simulink model "Exercicio_1_sim"  (R2016a)
settings: Solver=VariableStepAuto  StartTime=0.0  StopTime=t_sim  RelTol=1e-3
values from neighbouring files (symbols this model uses):
  A = [[0,1,0];[0,0,1];[-0.005,-0.11,-0.7]]    [Exercicio_1.m]    (also in matlab.mat = [0  1  0; 0  0  1; -0.005  -0.11  -0.7])
  A2 = [[-0.2,-0.2,0.4];[0.5,0,1];[0,-0.4,-0.4]]    [Exercicio_1.m]    (also in matlab.mat = [-0.2  -0.2  0.4; 0.5  0  1; 0  -0.4  -0.4])
  Aobs_A1 = A    [Exercicio_1.m]    (also in matlab.mat = [0  1  0; 0  0  1; -0.005  -0.11  -0.7])
  Aobs_B1 = A2    [Exercicio_1.m]    (also in matlab.mat = [-0.2  -0.2  0.4; 0.5  0  1; 0  -0.4  -0.4])
  B = [[0.1];[-0.2];[-0.1]]    [Exercicio_1.m]    (also in matlab.mat = [0.1 -0.2 -0.1])
  B2 = [[0.01];[0];[0.05]]    [Exercicio_1.m]    (also in matlab.mat = [0.01 0 0.05])
  Bobs_A1 = B    [Exercicio_1.m]    (also in matlab.mat = [0.1 -0.2 -0.1])
  Bobs_B1 = B2    [Exercicio_1.m]    (also in matlab.mat = [0.01 0 0.05])
  C = [0,0,1]    [Exercicio_1.m]    (also in matlab.mat = [0 0 1])
  C2 = [1,0,0]    [Exercicio_1.m]    (also in matlab.mat = [1 0 0])
  Cobs_A1 = C    [Exercicio_1.m]    (also in matlab.mat = [0 0 1])
  Cobs_B1 = C2    [Exercicio_1.m]    (also in matlab.mat = [1 0 0])
  D = [0]    [Exercicio_1.m]    (also in matlab.mat = 0)
  D2 = [0]    [Exercicio_1.m]    (also in matlab.mat = 0)
  Dobs_A1 = D    [Exercicio_1.m]    (also in matlab.mat = 0)
  Dobs_B1 = D2    [Exercicio_1.m]    (also in matlab.mat = 0)
  Keobs_A1 = [(Ke1_A1);(Ke2_A1);(Ke3_A1)]    [Exercicio_1.m]    (also in matlab.mat = [87026 -4185 9.81])
  Keobs_B1 = [(Ke1_B1);(Ke2_B1);(Ke3_B1)]    [Exercicio_1.m]    (also in matlab.mat = [8.18 -42.462 15.264])
settings Model: Creator=Usuario  LastModifiedBy=Eletrônica Auto Poli

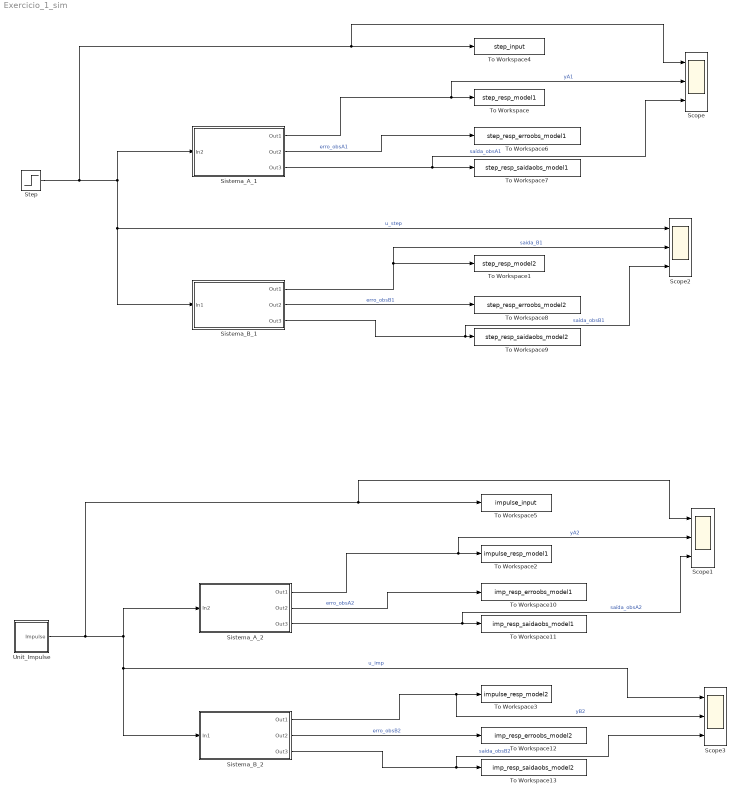
== system Exercicio_1_sim ==
  Scope{,1..3} (4 alike) : Scope  NumInputPorts=3
  Sistema_A_1 : Subsystem
  Sistema_A_2 : Subsystem
  Sistema_B_1 : Subsystem
  Sistema_B_2 : Subsystem
  Step : Step  SampleTime=0.01
  To Workspace : ToWorkspace  VariableName=step_resp_model1  SaveFormat=Timeseries  SampleTime=-1
  To Workspace1 : ToWorkspace  VariableName=step_resp_model2  SaveFormat=Timeseries  SampleTime=-1
  To Workspace10 : ToWorkspace  VariableName=imp_resp_erroobs_model1  SaveFormat=Timeseries  SampleTime=-1
  To Workspace11 : ToWorkspace  VariableName=imp_resp_saidaobs_model1  SaveFormat=Timeseries  SampleTime=-1
  To Workspace12 : ToWorkspace  VariableName=imp_resp_erroobs_model2  SaveFormat=Timeseries  SampleTime=-1
  To Workspace13 : ToWorkspace  VariableName=imp_resp_saidaobs_model2  SaveFormat=Timeseries  SampleTime=-1
  To Workspace2 : ToWorkspace  VariableName=impulse_resp_model1  SaveFormat=Timeseries  SampleTime=-1
  To Workspace3 : ToWorkspace  VariableName=impulse_resp_model2  SaveFormat=Timeseries  SampleTime=-1
  To Workspace4 : ToWorkspace  VariableName=step_input  SaveFormat=Timeseries  SampleTime=-1
  To Workspace5 : ToWorkspace  VariableName=impulse_input  SaveFormat=Timeseries  SampleTime=-1
  To Workspace6 : ToWorkspace  VariableName=step_resp_erroobs_model1  SaveFormat=Timeseries  SampleTime=-1
  To Workspace7 : ToWorkspace  VariableName=step_resp_saidaobs_model1  SaveFormat=Timeseries  SampleTime=-1
  To Workspace8 : ToWorkspace  VariableName=step_resp_erroobs_model2  SaveFormat=Timeseries  SampleTime=-1
  To Workspace9 : ToWorkspace  VariableName=step_resp_saidaobs_model2  SaveFormat=Timeseries  SampleTime=-1
  Unit_Impulse : Subsystem
  wires:
  Step/1 -> Scope/1, To Workspace4/1, Sistema_A_1/1(In2), Scope2/1, Sistema_B_1/1(In1)  "u_step"
  Sistema_A_1/1(Out1) -> Scope/2, To Workspace/1  "yA1"
  Sistema_A_1/2(Out2) -> To Workspace6/1  "erro_obsA1"
  Sistema_A_1/3(Out3) -> Scope/3, To Workspace7/1  "saída_obsA1"
  Sistema_B_1/2(Out2) -> To Workspace8/1  "erro_obsB1"
  Unit_Impulse/1(Impulse) -> Scope1/1, To Workspace5/1, Sistema_A_2/1(In2), Scope3/1, Sistema_B_2/1(In1)  "u_imp"
  Sistema_A_2/1(Out1) -> Scope1/2, To Workspace2/1  "yA2"
  Sistema_B_2/1(Out1) -> Scope3/2, To Workspace3/1  "yB2"
  Sistema_A_2/2(Out2) -> To Workspace10/1  "erro_obsA2"
  Sistema_A_2/3(Out3) -> Scope1/3, To Workspace11/1  "saída_obsA2"
  Sistema_B_2/2(Out2) -> To Workspace12/1  "erro_obsB2"
  Sistema_B_2/3(Out3) -> Scope3/3, To Workspace13/1  "saída_obsB2"
  Sistema_B_1/1(Out1) -> To Workspace1/1, Scope2/2  "saida_B1"
  Sistema_B_1/3(Out3) -> Scope2/3, To Workspace9/1  "saída_obsB1"

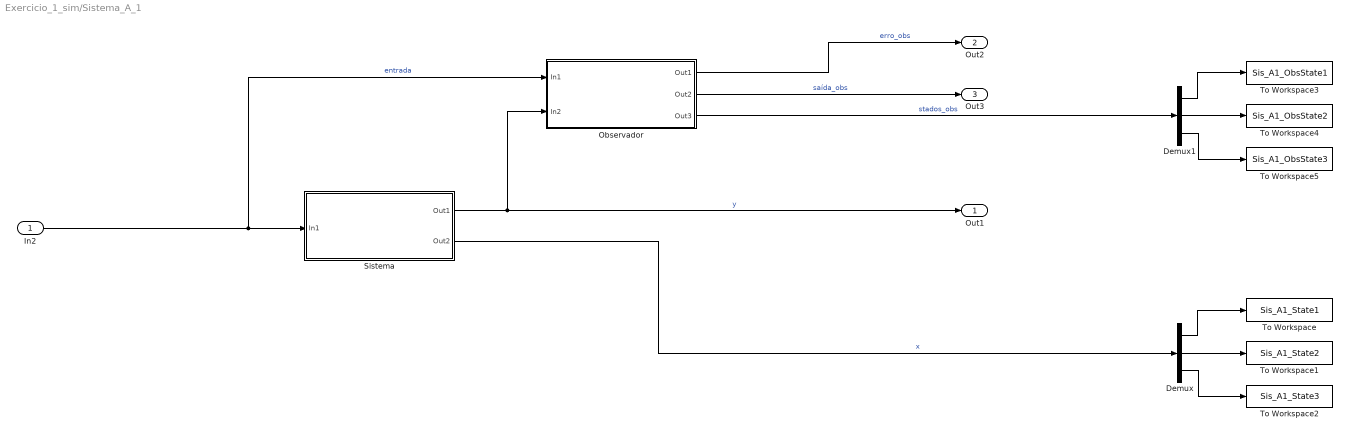
== system Exercicio_1_sim/Sistema_A_1 ==
  In2 : Inport
  Demux : Demux  Outputs=3
  Demux1 : Demux  Outputs=3
  Observador : Subsystem
  Sistema : Subsystem
  To Workspace : ToWorkspace  VariableName=Sis_A1_State1  SaveFormat=Timeseries  SampleTime=-1
  To Workspace1 : ToWorkspace  VariableName=Sis_A1_State2  SaveFormat=Timeseries  SampleTime=-1
  To Workspace2 : ToWorkspace  VariableName=Sis_A1_State3  SaveFormat=Timeseries  SampleTime=-1
  To Workspace3 : ToWorkspace  VariableName=Sis_A1_ObsState1  SaveFormat=Timeseries  SampleTime=-1
  To Workspace4 : ToWorkspace  VariableName=Sis_A1_ObsState2  SaveFormat=Timeseries  SampleTime=-1
  To Workspace5 : ToWorkspace  VariableName=Sis_A1_ObsState3  SaveFormat=Timeseries  SampleTime=-1
  Out1 : Outport
  Out2 : Outport  Port=2
  Out3 : Outport  Port=3
  wires:
  Demux/1 -> To Workspace/1
  Demux/2 -> To Workspace1/1
  Demux/3 -> To Workspace2/1
  In2/1 -> Observador/1(In1), Sistema/1(In1)  "entrada"
  Sistema/1(Out1) -> Out1/1, Observador/2(In2)  "y"
  Sistema/2(Out2) -> Demux/1  "x"
  Demux1/1 -> To Workspace3/1
  Demux1/2 -> To Workspace4/1
  Demux1/3 -> To Workspace5/1
  Observador/1(Out1) -> Out2/1  "erro_obs"
  Observador/2(Out2) -> Out3/1  "saída_obs"
  Observador/3(Out3) -> Demux1/1  "stados_obs"

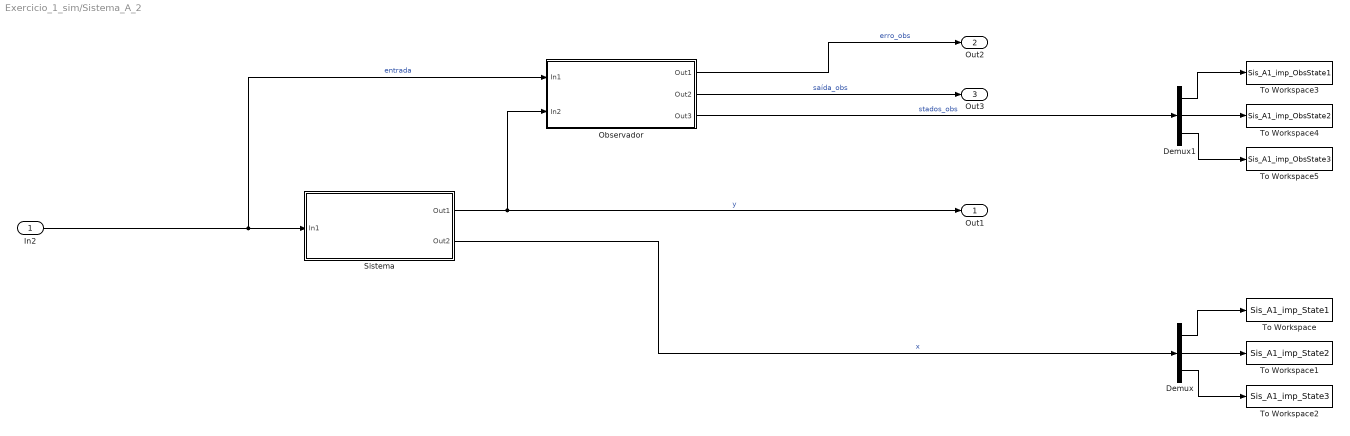
== system Exercicio_1_sim/Sistema_A_2 ==
  In2 : Inport
  Demux : Demux  Outputs=3
  Demux1 : Demux  Outputs=3
  Observador : Subsystem
  Sistema : Subsystem
  To Workspace : ToWorkspace  VariableName=Sis_A1_imp_State1  SaveFormat=Timeseries  SampleTime=-1
  To Workspace1 : ToWorkspace  VariableName=Sis_A1_imp_State2  SaveFormat=Timeseries  SampleTime=-1
  To Workspace2 : ToWorkspace  VariableName=Sis_A1_imp_State3  SaveFormat=Timeseries  SampleTime=-1
  To Workspace3 : ToWorkspace  VariableName=Sis_A1_imp_ObsState1  SaveFormat=Timeseries  SampleTime=-1
  To Workspace4 : ToWorkspace  VariableName=Sis_A1_imp_ObsState2  SaveFormat=Timeseries  SampleTime=-1
  To Workspace5 : ToWorkspace  VariableName=Sis_A1_imp_ObsState3  SaveFormat=Timeseries  SampleTime=-1
  Out1 : Outport
  Out2 : Outport  Port=2
  Out3 : Outport  Port=3
  wires:
  Demux/1 -> To Workspace/1
  Demux/2 -> To Workspace1/1
  Demux/3 -> To Workspace2/1
  In2/1 -> Observador/1(In1), Sistema/1(In1)  "entrada"
  Sistema/1(Out1) -> Out1/1, Observador/2(In2)  "y"
  Sistema/2(Out2) -> Demux/1  "x"
  Demux1/1 -> To Workspace3/1
  Demux1/2 -> To Workspace4/1
  Demux1/3 -> To Workspace5/1
  Observador/1(Out1) -> Out2/1  "erro_obs"
  Observador/2(Out2) -> Out3/1  "saída_obs"
  Observador/3(Out3) -> Demux1/1  "stados_obs"

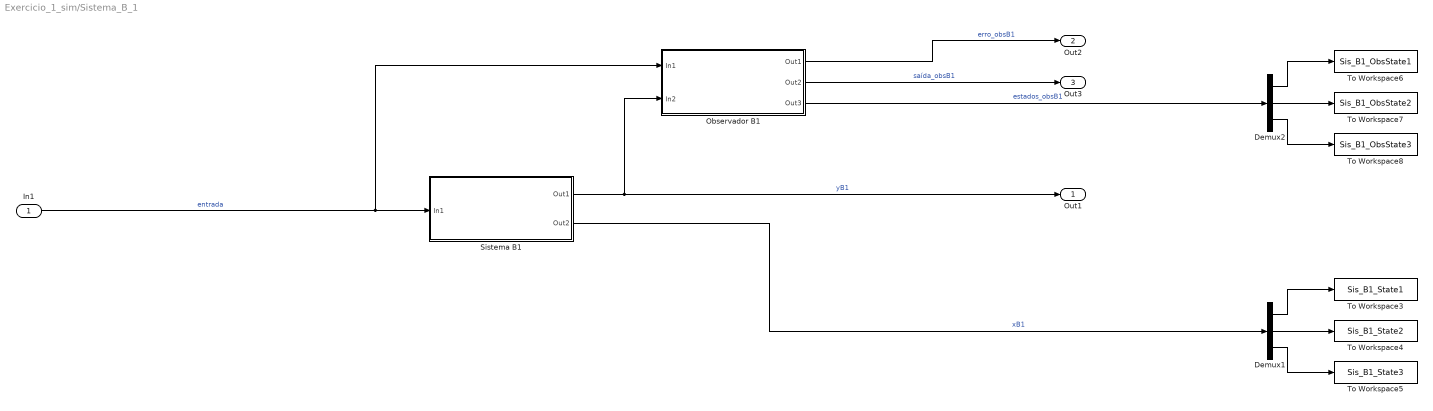
== system Exercicio_1_sim/Sistema_B_1 ==
  In1 : Inport
  Demux1 : Demux  Outputs=3
  Demux2 : Demux  Outputs=3
  Observador B1 : Subsystem
  Sistema B1 : Subsystem
  To Workspace3 : ToWorkspace  VariableName=Sis_B1_State1  SaveFormat=Timeseries  SampleTime=-1
  To Workspace4 : ToWorkspace  VariableName=Sis_B1_State2  SaveFormat=Timeseries  SampleTime=-1
  To Workspace5 : ToWorkspace  VariableName=Sis_B1_State3  SaveFormat=Timeseries  SampleTime=-1
  To Workspace6 : ToWorkspace  VariableName=Sis_B1_ObsState1  SaveFormat=Timeseries  SampleTime=-1
  To Workspace7 : ToWorkspace  VariableName=Sis_B1_ObsState2  SaveFormat=Timeseries  SampleTime=-1
  To Workspace8 : ToWorkspace  VariableName=Sis_B1_ObsState3  SaveFormat=Timeseries  SampleTime=-1
  Out1 : Outport
  Out2 : Outport  Port=2
  Out3 : Outport  Port=3
  wires:
  Demux1/1 -> To Workspace3/1
  Demux1/2 -> To Workspace4/1
  Demux1/3 -> To Workspace5/1
  In1/1 -> Observador B1/1(In1), Sistema B1/1(In1)  "entrada"
  Sistema B1/1(Out1) -> Out1/1, Observador B1/2(In2)  "yB1"
  Sistema B1/2(Out2) -> Demux1/1  "xB1"
  Demux2/1 -> To Workspace6/1
  Demux2/2 -> To Workspace7/1
  Demux2/3 -> To Workspace8/1
  Observador B1/1(Out1) -> Out2/1  "erro_obsB1"
  Observador B1/2(Out2) -> Out3/1  "saída_obsB1"
  Observador B1/3(Out3) -> Demux2/1  "estados_obsB1"

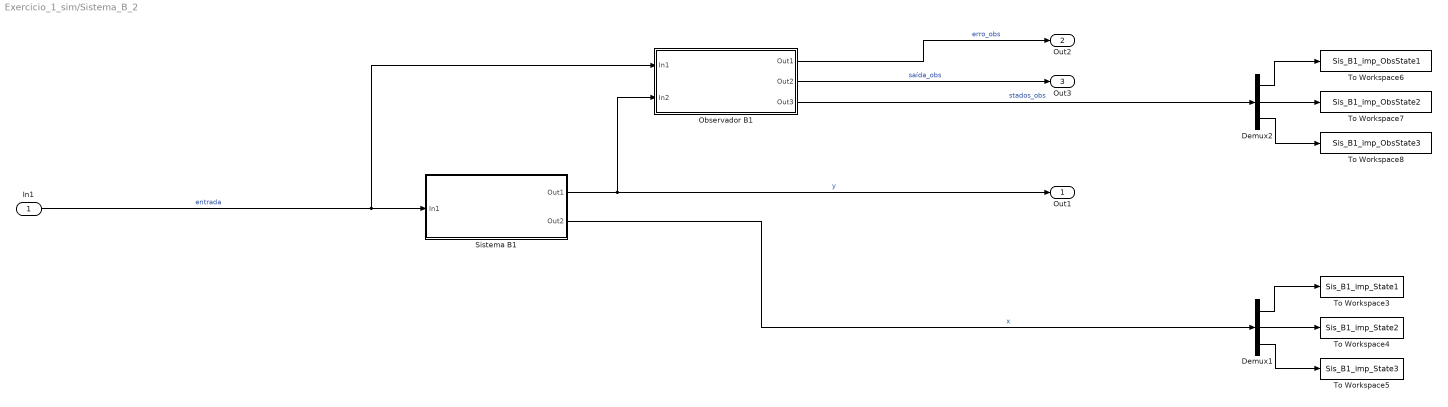
== system Exercicio_1_sim/Sistema_B_2 ==
  In1 : Inport
  Demux1 : Demux  Outputs=3
  Demux2 : Demux  Outputs=3
  Observador B1 : Subsystem
  Sistema B1 : Subsystem
  To Workspace3 : ToWorkspace  VariableName=Sis_B1_imp_State1  SaveFormat=Timeseries  SampleTime=-1
  To Workspace4 : ToWorkspace  VariableName=Sis_B1_imp_State2  SaveFormat=Timeseries  SampleTime=-1
  To Workspace5 : ToWorkspace  VariableName=Sis_B1_imp_State3  SaveFormat=Timeseries  SampleTime=-1
  To Workspace6 : ToWorkspace  VariableName=Sis_B1_imp_ObsState1  SaveFormat=Timeseries  SampleTime=-1
  To Workspace7 : ToWorkspace  VariableName=Sis_B1_imp_ObsState2  SaveFormat=Timeseries  SampleTime=-1
  To Workspace8 : ToWorkspace  VariableName=Sis_B1_imp_ObsState3  SaveFormat=Timeseries  SampleTime=-1
  Out1 : Outport
  Out2 : Outport  Port=2
  Out3 : Outport  Port=3
  wires:
  Demux1/1 -> To Workspace3/1
  Demux1/2 -> To Workspace4/1
  Demux1/3 -> To Workspace5/1
  In1/1 -> Observador B1/1(In1), Sistema B1/1(In1)  "entrada"
  Sistema B1/1(Out1) -> Out1/1, Observador B1/2(In2)  "y"
  Sistema B1/2(Out2) -> Demux1/1  "x"
  Demux2/1 -> To Workspace6/1
  Demux2/2 -> To Workspace7/1
  Demux2/3 -> To Workspace8/1
  Observador B1/1(Out1) -> Out2/1  "erro_obs"
  Observador B1/2(Out2) -> Out3/1  "saída_obs"
  Observador B1/3(Out3) -> Demux2/1  "stados_obs"

== system Exercicio_1_sim/Unit_Impulse ==
  Step1 : Step  Time=0.5  After=100  SampleTime=0.01
  Step2 : Step  Time=0.51  After=100  SampleTime=0.01
  Sum : Sum  Inputs=|+-
  Impulse : Outport
  wires:
  Step2/1 -> Sum/2
  Step1/1 -> Sum/1
  Sum/1 -> Impulse/1

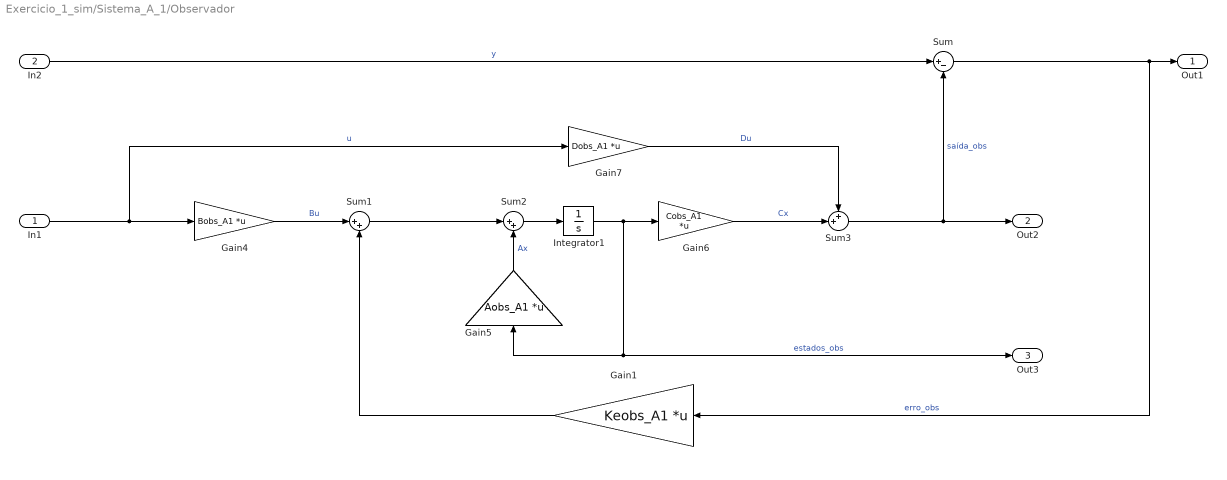
== system Exercicio_1_sim/Sistema_A_1/Observador ==
  In1 : Inport
  In2 : Inport  Port=2
  Gain1 : Gain  Gain=Keobs_A1  Multiplication=Matrix(K*u)
  Gain4 : Gain  Gain=Bobs_A1  Multiplication=Matrix(K*u)
  Gain5 : Gain  Gain=Aobs_A1  Multiplication=Matrix(K*u)
  Gain6 : Gain  Gain=Cobs_A1  Multiplication=Matrix(K*u)
  Gain7 : Gain  Gain=Dobs_A1  Multiplication=Matrix(K*u)
  Integrator1 : Integrator  InitialCondition=[3,7,5]
  Sum : Sum  Inputs=|+-
  Sum1 : Sum  Inputs=|++
  Sum2 : Sum  Inputs=|++
  Sum3 : Sum  Inputs=++|
  Out1 : Outport
  Out2 : Outport  Port=2
  Out3 : Outport  Port=3
  wires:
  Sum3/1 -> Out2/1, Sum/2  "saída_obs"
  Integrator1/1 -> Out3/1, Gain5/1, Gain6/1  "estados_obs"
  Gain6/1 -> Sum3/2  "Cx"
  Gain7/1 -> Sum3/1  "Du"
  Gain4/1 -> Sum1/1  "Bu"
  Gain5/1 -> Sum2/2  "Ax"
  Sum2/1 -> Integrator1/1
  In2/1 -> Sum/1  "y"
  In1/1 -> Gain4/1, Gain7/1  "u"
  Sum/1 -> Out1/1, Gain1/1  "erro_obs"
  Sum1/1 -> Sum2/1
  Gain1/1 -> Sum1/2

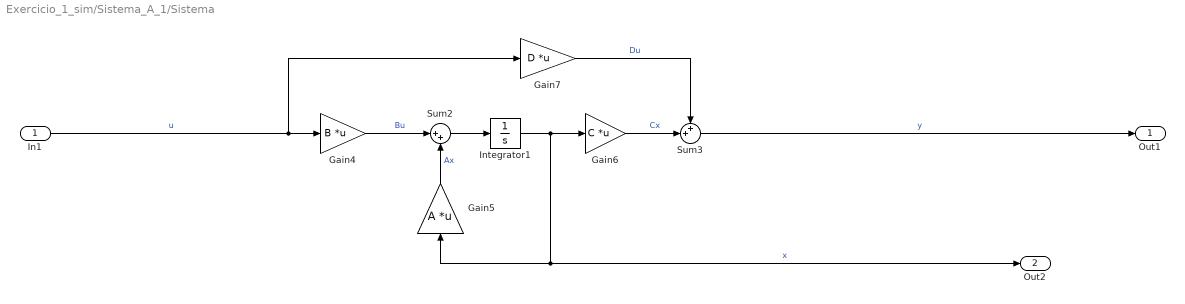
== system Exercicio_1_sim/Sistema_A_1/Sistema ==
  In1 : Inport
  Gain4 : Gain  Gain=B  Multiplication=Matrix(K*u)
  Gain5 : Gain  Gain=A  Multiplication=Matrix(K*u)
  Gain6 : Gain  Gain=C  Multiplication=Matrix(K*u)
  Gain7 : Gain  Gain=D  Multiplication=Matrix(K*u)
  Integrator1 : Integrator
  Sum2 : Sum  Inputs=|++
  Sum3 : Sum  Inputs=++|
  Out1 : Outport
  Out2 : Outport  Port=2
  wires:
  In1/1 -> Gain7/1, Gain4/1  "u"
  Sum3/1 -> Out1/1  "y"
  Integrator1/1 -> Out2/1, Gain5/1, Gain6/1  "x"
  Gain6/1 -> Sum3/2  "Cx"
  Gain7/1 -> Sum3/1  "Du"
  Gain4/1 -> Sum2/1  "Bu"
  Gain5/1 -> Sum2/2  "Ax"
  Sum2/1 -> Integrator1/1

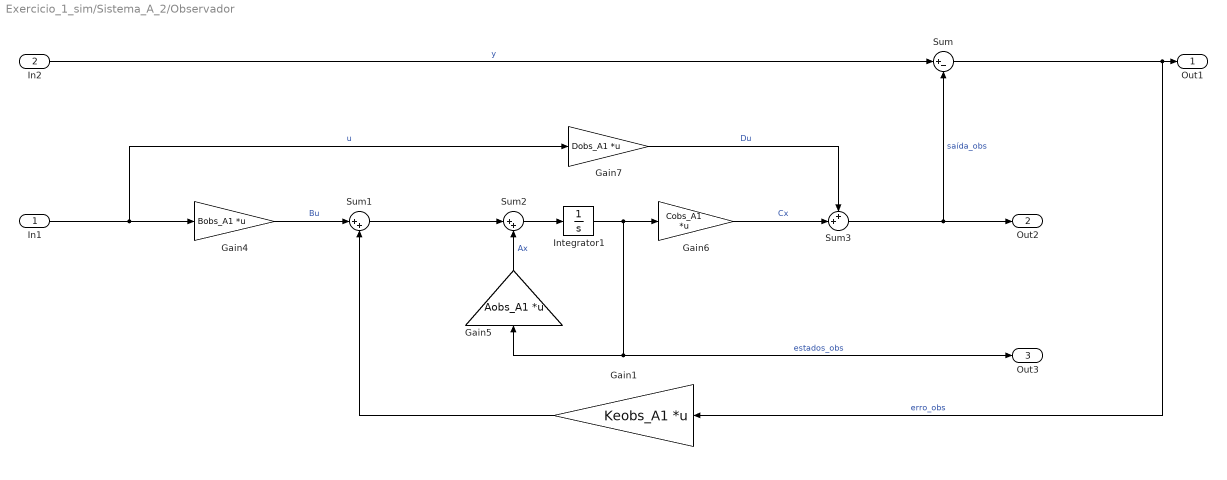
== system Exercicio_1_sim/Sistema_A_2/Observador ==
  In1 : Inport
  In2 : Inport  Port=2
  Gain1 : Gain  Gain=Keobs_A1  Multiplication=Matrix(K*u)
  Gain4 : Gain  Gain=Bobs_A1  Multiplication=Matrix(K*u)
  Gain5 : Gain  Gain=Aobs_A1  Multiplication=Matrix(K*u)
  Gain6 : Gain  Gain=Cobs_A1  Multiplication=Matrix(K*u)
  Gain7 : Gain  Gain=Dobs_A1  Multiplication=Matrix(K*u)
  Integrator1 : Integrator  InitialCondition=[7,9,13]
  Sum : Sum  Inputs=|+-
  Sum1 : Sum  Inputs=|++
  Sum2 : Sum  Inputs=|++
  Sum3 : Sum  Inputs=++|
  Out1 : Outport
  Out2 : Outport  Port=2
  Out3 : Outport  Port=3
  wires:
  Sum3/1 -> Out2/1, Sum/2  "saída_obs"
  Integrator1/1 -> Out3/1, Gain5/1, Gain6/1  "estados_obs"
  Gain6/1 -> Sum3/2  "Cx"
  Gain7/1 -> Sum3/1  "Du"
  Gain4/1 -> Sum1/1  "Bu"
  Gain5/1 -> Sum2/2  "Ax"
  Sum2/1 -> Integrator1/1
  In2/1 -> Sum/1  "y"
  In1/1 -> Gain4/1, Gain7/1  "u"
  Sum/1 -> Out1/1, Gain1/1  "erro_obs"
  Sum1/1 -> Sum2/1
  Gain1/1 -> Sum1/2

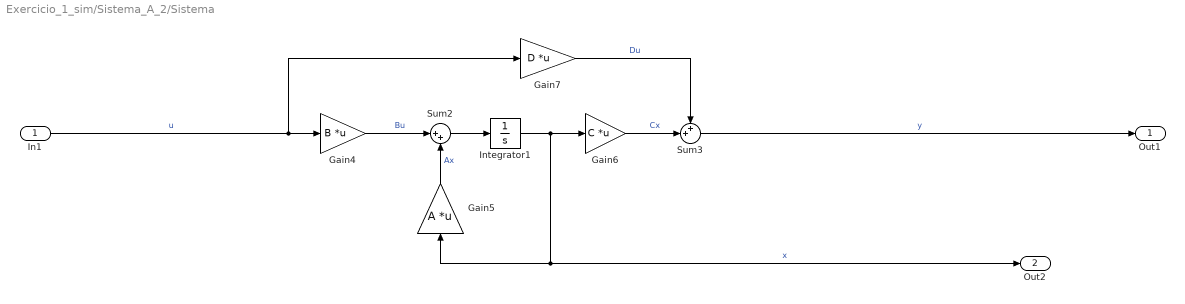
== system Exercicio_1_sim/Sistema_A_2/Sistema ==
  In1 : Inport
  Gain4 : Gain  Gain=B  Multiplication=Matrix(K*u)
  Gain5 : Gain  Gain=A  Multiplication=Matrix(K*u)
  Gain6 : Gain  Gain=C  Multiplication=Matrix(K*u)
  Gain7 : Gain  Gain=D  Multiplication=Matrix(K*u)
  Integrator1 : Integrator
  Sum2 : Sum  Inputs=|++
  Sum3 : Sum  Inputs=++|
  Out1 : Outport
  Out2 : Outport  Port=2
  wires:
  In1/1 -> Gain7/1, Gain4/1  "u"
  Sum3/1 -> Out1/1  "y"
  Integrator1/1 -> Out2/1, Gain5/1, Gain6/1  "x"
  Gain6/1 -> Sum3/2  "Cx"
  Gain7/1 -> Sum3/1  "Du"
  Gain4/1 -> Sum2/1  "Bu"
  Gain5/1 -> Sum2/2  "Ax"
  Sum2/1 -> Integrator1/1

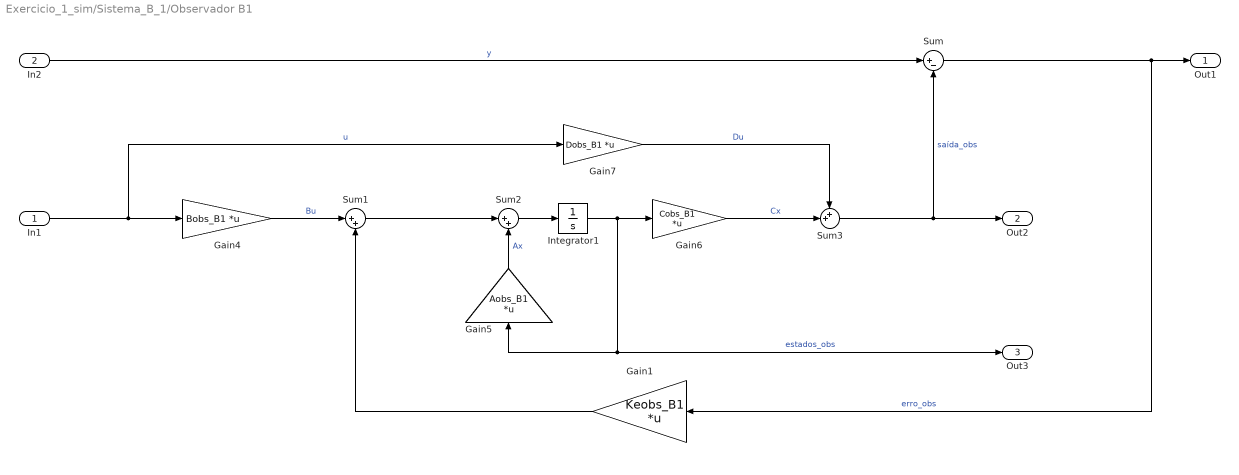
== system Exercicio_1_sim/Sistema_B_1/Observador B1 ==
  In1 : Inport
  In2 : Inport  Port=2
  Gain1 : Gain  Gain=Keobs_B1  Multiplication=Matrix(K*u)
  Gain4 : Gain  Gain=Bobs_B1  Multiplication=Matrix(K*u)
  Gain5 : Gain  Gain=Aobs_B1  Multiplication=Matrix(K*u)
  Gain6 : Gain  Gain=Cobs_B1  Multiplication=Matrix(K*u)
  Gain7 : Gain  Gain=Dobs_B1  Multiplication=Matrix(K*u)
  Integrator1 : Integrator  InitialCondition=[7,11,15]
  Sum : Sum  Inputs=|+-
  Sum1 : Sum  Inputs=|++
  Sum2 : Sum  Inputs=|++
  Sum3 : Sum  Inputs=++|
  Out1 : Outport
  Out2 : Outport  Port=2
  Out3 : Outport  Port=3
  wires:
  Sum3/1 -> Out2/1, Sum/2  "saída_obs"
  Integrator1/1 -> Out3/1, Gain5/1, Gain6/1  "estados_obs"
  Gain6/1 -> Sum3/2  "Cx"
  Gain7/1 -> Sum3/1  "Du"
  Gain4/1 -> Sum1/1  "Bu"
  Gain5/1 -> Sum2/2  "Ax"
  Sum2/1 -> Integrator1/1
  In2/1 -> Sum/1  "y"
  In1/1 -> Gain4/1, Gain7/1  "u"
  Sum/1 -> Out1/1, Gain1/1  "erro_obs"
  Sum1/1 -> Sum2/1
  Gain1/1 -> Sum1/2

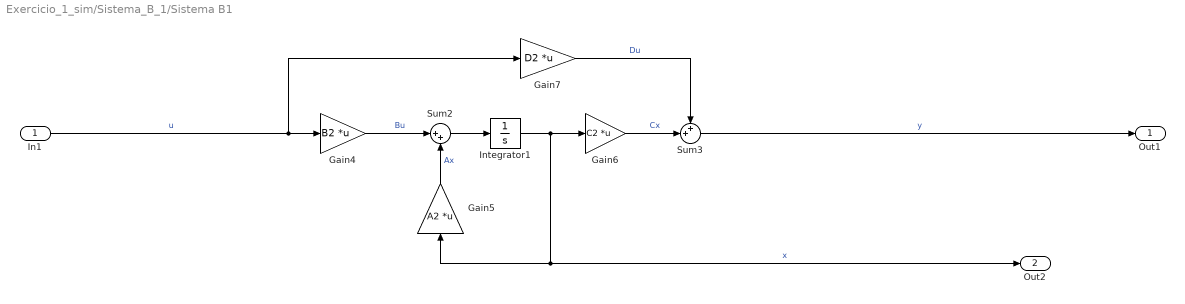
== system Exercicio_1_sim/Sistema_B_1/Sistema B1 ==
  In1 : Inport
  Gain4 : Gain  Gain=B2  Multiplication=Matrix(K*u)
  Gain5 : Gain  Gain=A2  Multiplication=Matrix(K*u)
  Gain6 : Gain  Gain=C2  Multiplication=Matrix(K*u)
  Gain7 : Gain  Gain=D2  Multiplication=Matrix(K*u)
  Integrator1 : Integrator
  Sum2 : Sum  Inputs=|++
  Sum3 : Sum  Inputs=++|
  Out1 : Outport
  Out2 : Outport  Port=2
  wires:
  In1/1 -> Gain7/1, Gain4/1  "u"
  Sum3/1 -> Out1/1  "y"
  Integrator1/1 -> Out2/1, Gain5/1, Gain6/1  "x"
  Gain6/1 -> Sum3/2  "Cx"
  Gain7/1 -> Sum3/1  "Du"
  Gain4/1 -> Sum2/1  "Bu"
  Gain5/1 -> Sum2/2  "Ax"
  Sum2/1 -> Integrator1/1

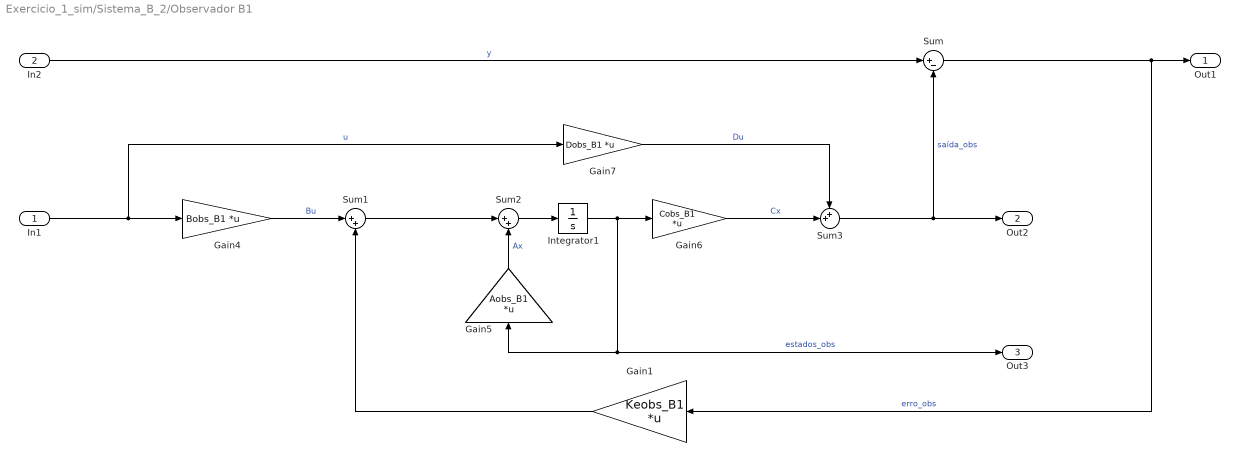
== system Exercicio_1_sim/Sistema_B_2/Observador B1 ==
  In1 : Inport
  In2 : Inport  Port=2
  Gain1 : Gain  Gain=Keobs_B1  Multiplication=Matrix(K*u)
  Gain4 : Gain  Gain=Bobs_B1  Multiplication=Matrix(K*u)
  Gain5 : Gain  Gain=Aobs_B1  Multiplication=Matrix(K*u)
  Gain6 : Gain  Gain=Cobs_B1  Multiplication=Matrix(K*u)
  Gain7 : Gain  Gain=Dobs_B1  Multiplication=Matrix(K*u)
  Integrator1 : Integrator  InitialCondition=[13,17,21]
  Sum : Sum  Inputs=|+-
  Sum1 : Sum  Inputs=|++
  Sum2 : Sum  Inputs=|++
  Sum3 : Sum  Inputs=++|
  Out1 : Outport
  Out2 : Outport  Port=2
  Out3 : Outport  Port=3
  wires:
  Sum3/1 -> Out2/1, Sum/2  "saída_obs"
  Integrator1/1 -> Out3/1, Gain5/1, Gain6/1  "estados_obs"
  Gain6/1 -> Sum3/2  "Cx"
  Gain7/1 -> Sum3/1  "Du"
  Gain4/1 -> Sum1/1  "Bu"
  Gain5/1 -> Sum2/2  "Ax"
  Sum2/1 -> Integrator1/1
  In2/1 -> Sum/1  "y"
  In1/1 -> Gain4/1, Gain7/1  "u"
  Sum/1 -> Out1/1, Gain1/1  "erro_obs"
  Sum1/1 -> Sum2/1
  Gain1/1 -> Sum1/2

== system Exercicio_1_sim/Sistema_B_2/Sistema B1 ==
  In1 : Inport
  Gain4 : Gain  Gain=B2  Multiplication=Matrix(K*u)
  Gain5 : Gain  Gain=A2  Multiplication=Matrix(K*u)
  Gain6 : Gain  Gain=C2  Multiplication=Matrix(K*u)
  Gain7 : Gain  Gain=D2  Multiplication=Matrix(K*u)
  Integrator1 : Integrator
  Sum2 : Sum  Inputs=|++
  Sum3 : Sum  Inputs=++|
  Out1 : Outport
  Out2 : Outport  Port=2
  wires:
  In1/1 -> Gain7/1, Gain4/1  "u"
  Sum3/1 -> Out1/1  "y"
  Integrator1/1 -> Out2/1, Gain5/1, Gain6/1  "x"
  Gain6/1 -> Sum3/2  "Cx"
  Gain7/1 -> Sum3/1  "Du"
  Gain4/1 -> Sum2/1  "Bu"
  Gain5/1 -> Sum2/2  "Ax"
  Sum2/1 -> Integrator1/1
